simulink model "audio"  (R2024b)
settings: Solver=FixedStepAuto  StartTime=0.0  StopTime=10.0  RelTol=1e-3
model workspace (MAT data in the model file):
  Password = Simulink.Parameter
  Password.Complexity = 'real'
  Password.Dimensions = [0 0]
  Password.DataType = 'auto'
undefined symbols (not defined in the file): Radix
libraries: androidsensorlib x2, dspxfrm3 x2, androidcommunicationlib x2, androidaudiovideolib x1, dspsigops x1
settings Model: Creator=hrida  LastModifiedBy=hrida
settings OptimizationCC: DefaultParameterBehavior=Inlined  EnhancedBackFolding=on  PassReuseOutputArgsAs=Individual arguments  ZeroExternalMemoryAtStartup=off  ZeroInternalMemoryAtStartup=off  MaxStackSize=64  OptimizeBlockOrder=speed  DifferentSizesBufferReuse=on  OptimizationCustomize=off  EfficientTunableParamExpr=on
settings DebuggingCC: ParameterTunabilityLossMsg=error
settings HardwareCC: ProdBitPerLong=64  ProdLargestAtomicInteger=LongLong  ProdLargestAtomicFloat=Double  ProdLongLongMode=on  ProdHWDeviceType=ARM Compatible->ARM Cortex-A (64-bit)
settings RTWCC: Description=Embedded Coder  SystemTargetFile=ert.tlc  HardwareBoard=Android Device (64bit)  TLCOptions="-aInlineSetEventsForThisBaseRateFcn=TLC_FALSE -aSuppressMultiTaskScheduler=TLC_FALSE  -aRateBasedStepFcn=0"  TemplateMakefile=ert_default_tmf  RTWVerbose=off  Toolchain=Android SDK/NDK Tools
settings CodeAppCC: ForceParamTrailComments=on  IgnoreCustomStorageClasses=off  OperatorAnnotations=on  SimulinkDataObjDesc=on  SFDataObjDesc=on  InsertBlockDesc=on
settings ERTTargetCC: SupportContinuousTime=on  SupportVariableSizeSignals=on

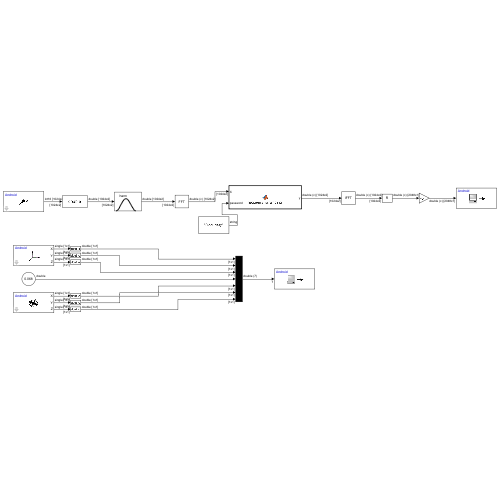
[thumbnail: Simulink's stored preview of the top-level diagram]
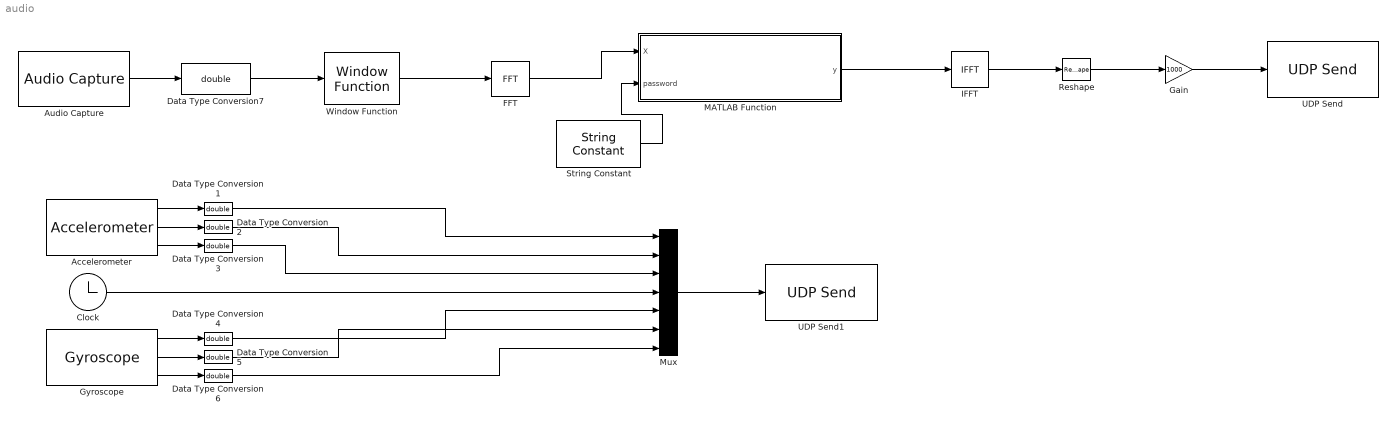
== system audio ==
  Accelerometer : androidsensorlib/Accelerometer  OutputVector=off  SampleTime=0.1  BlockPlatform=Android
  Audio Capture : androidaudiovideolib/Audio Capture  SampleFreq=16000  FrameSize=1024  SampleTime=0.064  SimulateUsing=Code generation  DeviceStr=0  QueueDuration=0  BlockPlatform=Android  AudioSamplingFreq=44100
  Clock : Clock
  Data Type Conversion{1..7} (7 alike) : DataTypeConversion  OutDataTypeStr=double  SaturateOnIntegerOverflow=off  RndMeth=Floor
  FFT : dspxfrm3/FFT  FFTImplementation=Radix-2  CompMethod=Table lookup  TableOpt=NEW  TableOptActive=Speed  BitRevOrder=off  Normalize=off  InheritFFTLength=on  FFTLength=64  WrapInput=on  roundingMode=Ceiling  overflowMode=off  firstCoeffDataTypeStr=Inherit: Same word length as input  firstCoeffLastDataTypeStr=Inherit: Same word length as input  outputMin=[]  outputMax=[]
      settings: LockScale=on
  Gain : Gain  Gain=1000
  Gyroscope : androidsensorlib/Gyroscope  OutputVector=off  SampleTime=0.1  BlockPlatform=Android
  IFFT : dspxfrm3/IFFT  FFTImplementation=Radix-2  CompMethod=Table lookup  TableOpt=NEW  TableOptActive=Speed  BitRevOrder=off  cs_in=off  Normalize=on  InheritFFTLength=on  FFTLength=64  WrapInput=on  mode=Real  outSamplingMode=Sample based  roundingMode=Ceiling  overflowMode=off  firstCoeffDataTypeStr=Inherit: Same word length as input  firstCoeffLastDataTypeStr=Inherit: Same word length as input  accumDataTypeStr=Inherit: Same as product output  accumLastDataTypeStr=Inherit: Same as product output  outputMin=[]  outputMax=[]
  MATLAB Function : MATLAB Function  TreatAsAtomicUnit=on
  Mux : Mux  Inputs=7
  Reshape : Reshape  OutputDimensionality=Customize  OutputDimensions=[2048,1]
  String Constant : StringConstant  String="\"Frequency\""
  UDP Send : androidcommunicationlib/UDP Send  remoteURL='10.7.5.118'  remotePort=25000  localURL='0.0.0.0'  localPortSource=Automatically determine  localPort=-1  sampletime=-1  blockPlatform=Android  separateLengthPort=0
  UDP Send1 : androidcommunicationlib/UDP Send  remoteURL='10.7.5.118'  remotePort=25001  localURL='0.0.0.0'  localPortSource=Automatically determine  localPort=-1  sampletime=-1  blockPlatform=Android  separateLengthPort=0
  Window Function : dspsigops/Window Function  winmode=Apply window to input  wintype=Hann  sampmode=Continuous  samptime=1  N=64  Rs=50  beta=10  winsamp=Symmetric  UserWindow=hamming  OptParams=off  UserParams={'symmetric'}  dataType=double  isSigned=on  wordLen=16  udDataType=sfix(16)  fracBitsMode=Best precision  numFracBits=15  roundingMode=Floor  overflowMode=off  numSidelobes=4  sidelobeLevel=-30
  wires:
  Window Function/1 -> FFT/1
  MATLAB Function/1(y) -> IFFT/1
  FFT/1 -> MATLAB Function/1(X)
  Mux/1 -> UDP Send1/1
  String Constant/1 -> MATLAB Function/2(password)
  Clock/1 -> Mux/4
  Accelerometer/1 -> Data Type Conversion1/1
  Accelerometer/2 -> Data Type Conversion2/1
  Accelerometer/3 -> Data Type Conversion3/1
  Gyroscope/2 -> Data Type Conversion5/1
  Gyroscope/1 -> Data Type Conversion4/1
  Gyroscope/3 -> Data Type Conversion6/1
  Data Type Conversion1/1 -> Mux/1
  Data Type Conversion2/1 -> Mux/2
  Data Type Conversion3/1 -> Mux/3
  Data Type Conversion4/1 -> Mux/5
  Data Type Conversion5/1 -> Mux/6
  Data Type Conversion6/1 -> Mux/7
  IFFT/1 -> Reshape/1
  Data Type Conversion7/1 -> Window Function/1
  Audio Capture/1 -> Data Type Conversion7/1
  Reshape/1 -> Gain/1
  Gain/1 -> UDP Send/1

== matlab function audio/MATLAB Function ==
  data: X input; y output; password input
function y = frequency_scrambling(X,password)

seed=sum(double(char(password)))+length(password);
rng(seed);
key=randperm(511)+1;

y=X;

y(1)=X(1); %DC
y(513)=X(513); %Nyquist

y(2:512)=X(key);
y(514:1024)=conj(flipud(y(2:512)));
end
